simulink subsystem "EnergyStorage"  (R2023b)
settings: Solver=VariableStepAuto  StartTime=0.0  StopTime=10.0  RelTol=1e-3
undefined symbols (not defined in the file): BESSoCReset, C1_LUT, C2_LUT, DiscIntNeverNeededParam, NCellsParallel, NCellsSeries, OCV_LUT, R0_LUT, R1_LUT, R2_LUT, rCellCapacity, rInitialSoC, SoC_BP, TCell_BP, tSimBattMgt
settings Model: DataDictionary=BatteryManagement_data.sldd  EnableAccessToBaseWorkspace=off  Creator=Elio  LastModifiedBy=Elio

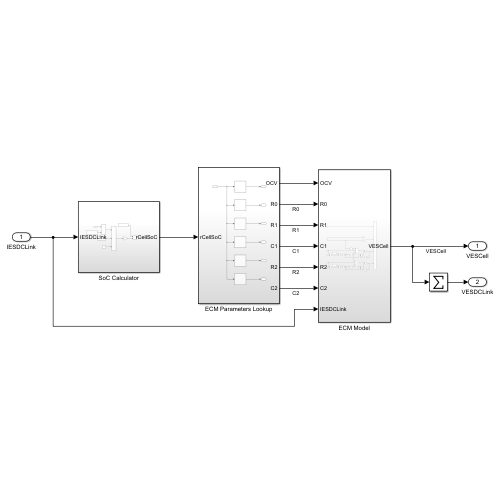
[thumbnail: Simulink's stored preview of the top-level diagram]
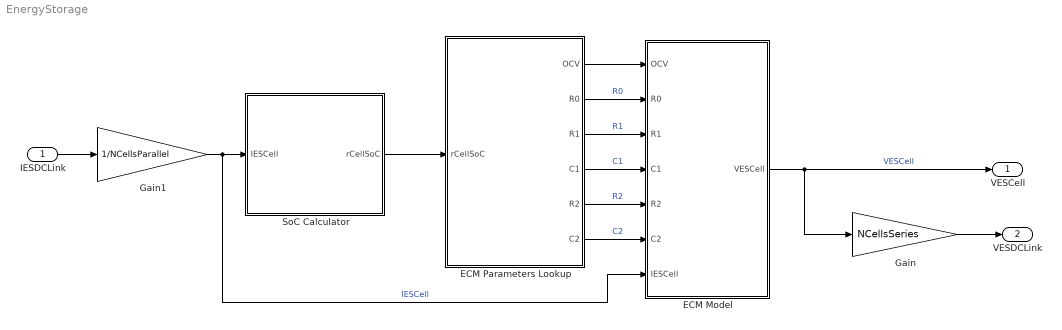
== system EnergyStorage ==
  IESDCLink : Inport
  ECM Model : Subsystem
  ECM Parameters Lookup : Subsystem
  Gain : Gain  Gain=NCellsSeries
  Gain1 : Gain  Gain=1/NCellsParallel
  SoC Calculator : Subsystem
  VESCell : Outport
  VESDCLink : Outport  Port=2
  wires:
  Gain/1 -> VESDCLink/1
  ECM Model/1(VESCell) -> VESCell/1, Gain/1  "VESCell"
  IESDCLink/1 -> Gain1/1
  ECM Parameters Lookup/2(R0) -> ECM Model/2(R0)  "R0"
  ECM Parameters Lookup/1(OCV) -> ECM Model/1(OCV)
  ECM Parameters Lookup/6(C2) -> ECM Model/6(C2)  "C2"
  SoC Calculator/1(rCellSoC) -> ECM Parameters Lookup/1(rCellSoC)
  ECM Parameters Lookup/4(C1) -> ECM Model/4(C1)  "C1"
  ECM Parameters Lookup/5(R2) -> ECM Model/5(R2)  "R2"
  ECM Parameters Lookup/3(R1) -> ECM Model/3(R1)  "R1"
  Gain1/1 -> SoC Calculator/1(IESCell), ECM Model/7(IESCell)  "IESCell"

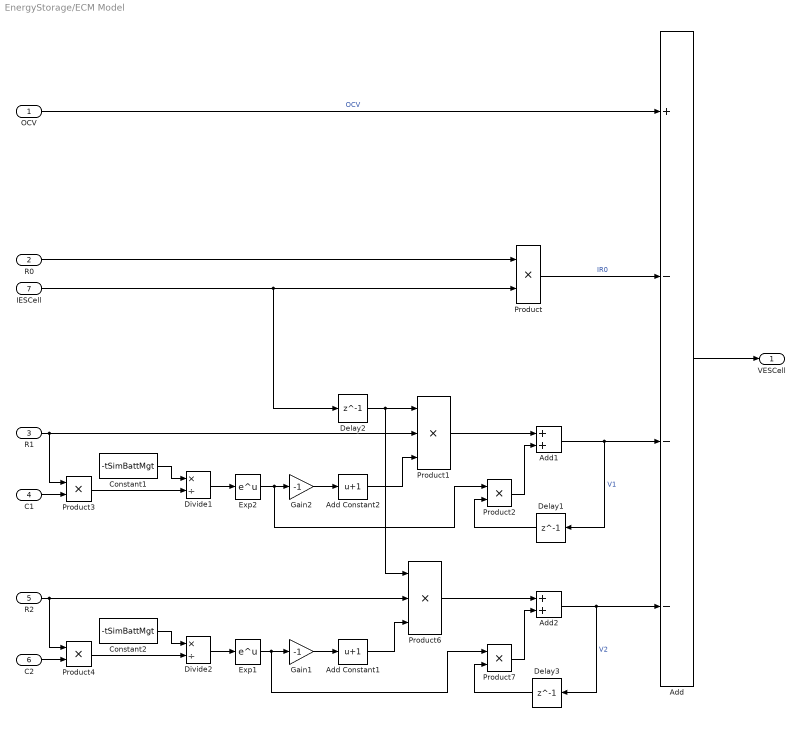
== system EnergyStorage/ECM Model ==
  OCV : Inport
  R0 : Inport  Port=2
  R1 : Inport  Port=3
  C1 : Inport  Port=4
  R2 : Inport  Port=5
  C2 : Inport  Port=6
  IESCell : Inport  Port=7
  Add : Sum  Inputs=+---
  Add Constant1 : Bias  Bias=1  SaturateOnIntegerOverflow=off
  Add Constant2 : Bias  Bias=1  SaturateOnIntegerOverflow=off
  Add1 : Sum
  Add2 : Sum
  Constant1 : Constant  Value=-tSimBattMgt  SampleTime=tSimBattMgt
  Constant2 : Constant  Value=-tSimBattMgt  SampleTime=tSimBattMgt
  Delay1 : Delay  DelayLength=1
  Delay2 : Delay  DelayLength=1
  Delay3 : Delay  DelayLength=1
  Divide1 : Product  Inputs=*/
  Divide2 : Product  Inputs=*/
  Exp1 : Math
  Exp2 : Math
  Gain1 : Gain  Gain=-1
  Gain2 : Gain  Gain=-1
  Product{,2..4,7} (5 alike) : Product
  Product1 : Product  Inputs=3
  Product6 : Product  Inputs=3
  VESCell : Outport
  wires:
  IESCell/1 -> Product/2, Delay2/1
  R0/1 -> Product/1
  OCV/1 -> Add/1  "OCV"
  Product/1 -> Add/2  "IR0"
  Add/1 -> VESCell/1
  Delay3/1 -> Product7/2
  Gain1/1 -> Add Constant1/1
  Divide2/1 -> Exp1/1
  Constant2/1 -> Divide2/1
  Exp1/1 -> Product7/1, Gain1/1
  Add2/1 -> Delay3/1, Add/4  "V2"
  Product6/1 -> Add2/1
  Add Constant1/1 -> Product6/3
  Product7/1 -> Add2/2
  Product1/1 -> Add1/1
  Delay1/1 -> Product2/2
  Product2/1 -> Add1/2
  Exp2/1 -> Product2/1, Gain2/1
  Constant1/1 -> Divide1/1
  Add1/1 -> Delay1/1, Add/3  "V1"
  Divide1/1 -> Exp2/1
  R1/1 -> Product3/1, Product1/2
  Add Constant2/1 -> Product1/3
  Gain2/1 -> Add Constant2/1
  C1/1 -> Product3/2
  Product3/1 -> Divide1/2
  Product4/1 -> Divide2/2
  C2/1 -> Product4/2
  R2/1 -> Product4/1, Product6/2
  Delay2/1 -> Product1/1, Product6/1

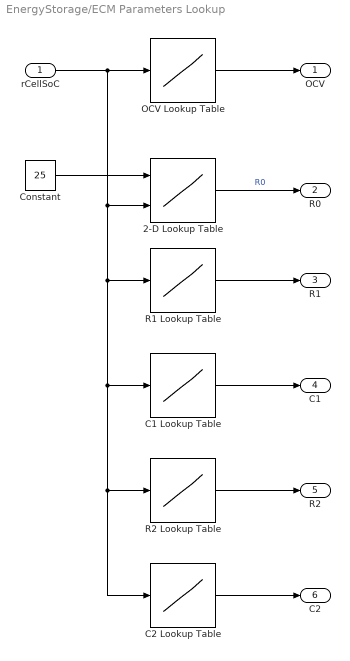
== system EnergyStorage/ECM Parameters Lookup ==
  rCellSoC : Inport
  2-D Lookup Table : Lookup_n-D  BreakpointsForDimension1=TCell_BP  BreakpointsForDimension2=SoC_BP  Table=R0_LUT  InternalRulePriority=Speed  RndMeth=Simplest
      settings: InputPortMap=u0,u1
  C1 Lookup Table : Lookup_n-D  NumberOfTableDimensions=1  LookupTableObject=''  BreakpointsForDimension1=SoC_BP  BreakpointsForDimension1FirstPoint=10  BreakpointsForDimension2FirstPoint=10  BreakpointsForDimension1Spacing=12  BreakpointsForDimension2Spacing=12  IndexSearchMethod=Evenly spaced points  Table=C1_LUT  DiagnosticForOutOfRangeInput=Error  InternalRulePriority=Speed  RndMeth=Simplest
  C2 Lookup Table : Lookup_n-D  NumberOfTableDimensions=1  LookupTableObject=''  BreakpointsForDimension1=SoC_BP  BreakpointsForDimension1FirstPoint=10  BreakpointsForDimension2FirstPoint=10  BreakpointsForDimension1Spacing=12  BreakpointsForDimension2Spacing=12  IndexSearchMethod=Evenly spaced points  Table=C2_LUT  DiagnosticForOutOfRangeInput=Error  InternalRulePriority=Speed  RndMeth=Simplest
  Constant : Constant  Value=25
  OCV Lookup Table : Lookup_n-D  NumberOfTableDimensions=1  LookupTableObject=''  BreakpointsForDimension1=SoC_BP  BreakpointsForDimension1FirstPoint=10  BreakpointsForDimension2FirstPoint=10  BreakpointsForDimension1Spacing=12  BreakpointsForDimension2Spacing=12  Table=OCV_LUT  DiagnosticForOutOfRangeInput=Error  InternalRulePriority=Speed  RndMeth=Simplest
  R1 Lookup Table : Lookup_n-D  NumberOfTableDimensions=1  LookupTableObject=''  BreakpointsForDimension1=SoC_BP  BreakpointsForDimension1FirstPoint=10  BreakpointsForDimension2FirstPoint=10  BreakpointsForDimension1Spacing=12  BreakpointsForDimension2Spacing=12  IndexSearchMethod=Evenly spaced points  Table=R1_LUT  DiagnosticForOutOfRangeInput=Error  InternalRulePriority=Speed  RndMeth=Simplest
  R2 Lookup Table : Lookup_n-D  NumberOfTableDimensions=1  LookupTableObject=''  BreakpointsForDimension1=SoC_BP  BreakpointsForDimension1FirstPoint=10  BreakpointsForDimension2FirstPoint=10  BreakpointsForDimension1Spacing=12  BreakpointsForDimension2Spacing=12  IndexSearchMethod=Evenly spaced points  Table=R2_LUT  DiagnosticForOutOfRangeInput=Error  InternalRulePriority=Speed  RndMeth=Simplest
  OCV : Outport
  R0 : Outport  Port=2
  R1 : Outport  Port=3
  C1 : Outport  Port=4
  R2 : Outport  Port=5
  C2 : Outport  Port=6
  wires:
  Constant/1 -> 2-D Lookup Table/1
  rCellSoC/1 -> R1 Lookup Table/1, C2 Lookup Table/1, R2 Lookup Table/1, C1 Lookup Table/1, 2-D Lookup Table/2, OCV Lookup Table/1
  OCV Lookup Table/1 -> OCV/1
  2-D Lookup Table/1 -> R0/1  "R0"
  R1 Lookup Table/1 -> R1/1
  C1 Lookup Table/1 -> C1/1
  R2 Lookup Table/1 -> R2/1
  C2 Lookup Table/1 -> C2/1

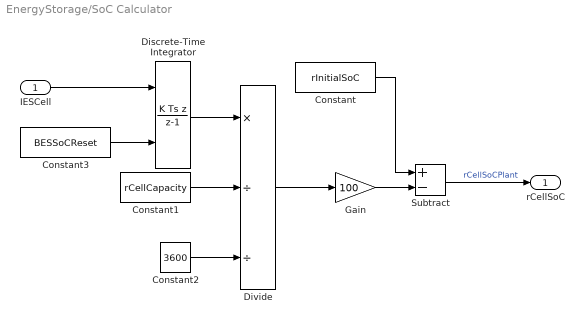
== system EnergyStorage/SoC Calculator ==
  IESCell : Inport
  Constant : Constant  Value=rInitialSoC  SampleTime=tSimBattMgt
  Constant1 : Constant  Value=rCellCapacity  SampleTime=tSimBattMgt
  Constant2 : Constant  Value=3600  SampleTime=tSimBattMgt
  Constant3 : Constant  Value=BESSoCReset  SampleTime=tSimBattMgt
  Discrete-Time Integrator : DiscreteIntegrator  IntegratorMethod=Integration: Backward Euler  ExternalReset=rising  SampleTime=-1  ICPrevOutput=DiscIntNeverNeededParam  ICPrevScaledInput=DiscIntNeverNeededParam
  Divide : Product  Inputs=*//
  Gain : Gain  Gain=100
  Subtract : Sum  Inputs=+-
  rCellSoC : Outport
  wires:
  IESCell/1 -> Discrete-Time Integrator/1
  Constant/1 -> Subtract/1
  Discrete-Time Integrator/1 -> Divide/1
  Constant1/1 -> Divide/2
  Divide/1 -> Gain/1
  Gain/1 -> Subtract/2
  Subtract/1 -> rCellSoC/1  "rCellSoCPlant"
  Constant2/1 -> Divide/3
  Constant3/1 -> Discrete-Time Integrator/2
